simulink model "Lab1Exp1Passo2"  (R2021a)
settings: Solver=FixedStepAuto  StartTime=0.0  StopTime=100  FixedStep=1e-5  RelTol=1e-3
values from neighbouring files (symbols this model uses):
  d = 0.6    [Lab1Exp1.m]    (also in Lab1Teste2.m)
  k1 = -1/L    (= -1000)    [Conversor.m]    (also in Lab1Exp1.m)
  k2 = rl*k1    (= 0)    [Conversor.m]    (also in Lab1Exp1.m)
  k3 = -Vin*k1    (= 20000)    [Conversor.m]    (also in Lab1Exp1.m)
  k4 = 1/C    (= 454.545454545)    [Conversor.m]    (also in Lab1Exp1.m)
  k5 = -k4/R    (= -113.636363636)    [Conversor.m]    (also in Lab1Exp1.m)
  k6 = k4*Po    (= 4545.45454545)    [Conversor.m]    (also in Lab1Exp1.m)
settings Model: Creator=DaniSan  LastModifiedBy=DaniSan

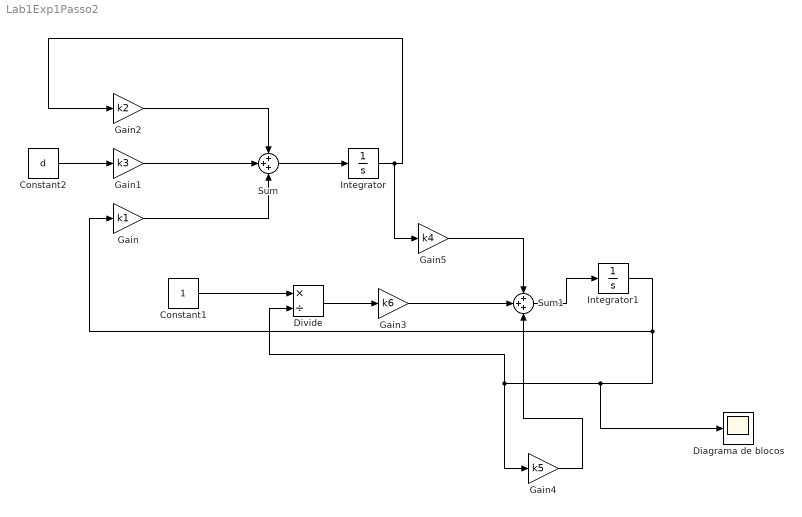
== system Lab1Exp1Passo2 ==
  Constant1 : Constant
  Constant2 : Constant  Value=d
  Diagrama de blocos : Scope
      settings: Tag=simout
  Divide : Product  Inputs=*/
  Gain : Gain  Gain=k1
  Gain1 : Gain  Gain=k3
  Gain2 : Gain  Gain=k2
  Gain3 : Gain  Gain=k6
  Gain4 : Gain  Gain=k5
  Gain5 : Gain  Gain=k4
  Integrator : Integrator  InitialCondition=0.0001
  Integrator1 : Integrator  InitialCondition=0.0001
  Sum : Sum  Inputs=+++
  Sum1 : Sum  Inputs=+++
  wires:
  Gain2/1 -> Sum/1
  Gain1/1 -> Sum/2
  Gain/1 -> Sum/3
  Sum/1 -> Integrator/1
  Integrator/1 -> Gain5/1, Gain2/1
  Gain5/1 -> Sum1/1
  Sum1/1 -> Integrator1/1
  Integrator1/1 -> Gain/1, Diagrama de blocos/1, Divide/2, Gain4/1
  Gain4/1 -> Sum1/3
  Gain3/1 -> Sum1/2
  Constant1/1 -> Divide/1
  Divide/1 -> Gain3/1
  Constant2/1 -> Gain1/1
